simulink model "Thrustersim"  (R2018b)
settings: Solver=FixedStepAuto  StartTime=0.0  StopTime=100.0  FixedStep=.1  RelTol=1e-3
values from neighbouring files (symbols this model uses):
  R_2_t = [1 1 -1 -1; 1 -1 -1 1; 1 -1 1 -1; 1 1 1 1]    [Thruster_supprt.m]
libraries: simulink x3
settings Model: DataTypeOverride=Double  MinMaxOverflowLogging=ForceOff  Creator=Stefan's Laptop  LastModifiedBy=Stefan's Laptop

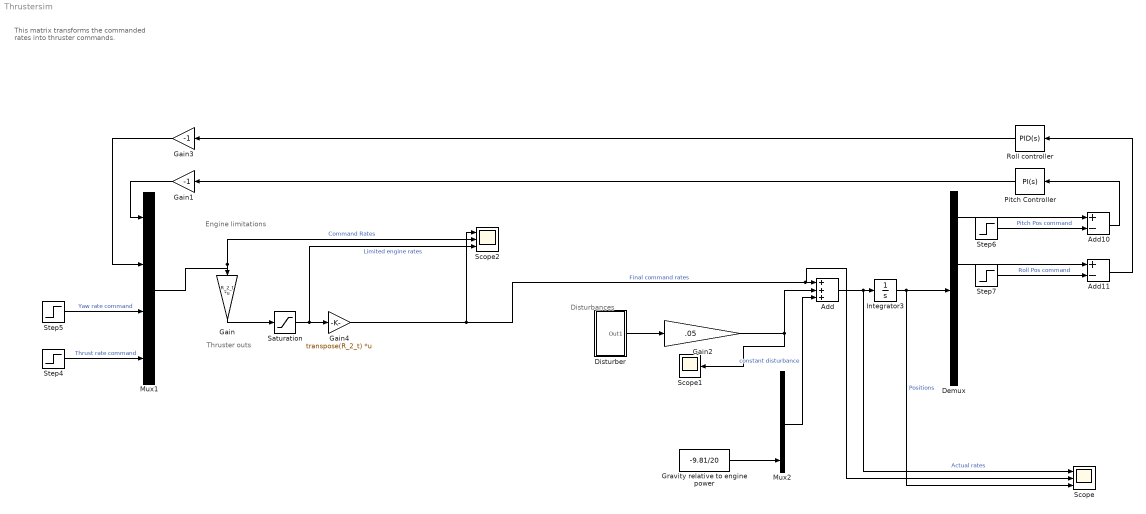
== system Thrustersim ==
  note: Engine limitations
  note: Disturbances
  note: Thruster outs
  note: This matrix transforms the commanded
      | rates into thruster commands.
  Add : Sum  Inputs=3
  Add10 : Sum  Inputs=+-
  Add11 : Sum  Inputs=+-
  Demux : Demux
  Disturber : Subsystem
  Gain : Gain  Gain=R_2_t  Multiplication=Matrix(K*u)
  Gain1 : Gain  Gain=-1
  Gain2 : Gain  Gain=.05
  Gain3 : Gain  Gain=-1
  Gain4 : Gain  Gain=transpose(R_2_t)  Multiplication=Matrix(K*u)
  Gravity relative to engine power : Constant  Value=-9.81/20
  Integrator3 : Integrator
  Mux1 : Mux
  Mux2 : Mux
  Pitch Controller : simulink/Continuous/PID Controller  Controller=PI  Form=Parallel  TimeDomain=Continuous-time  SampleTime=-1  IntegratorMethod=Forward Euler  FilterMethod=Forward Euler  ControllerParametersSource=internal  P=1  I=200  D=1  UseFilter=on  N=100  TunerSelectOption=Transfer Function Based (PID Tuner App)  InitialConditionSource=internal  InitialConditionForIntegrator=0  InitialConditionForFilter=0  DifferentiatorICPrevScaledInput=0  ExternalReset=none  TrackingMode=off  Kt=1  LimitOutput=off  UpperSaturationLimit=inf  LowerSaturationLimit=-inf  LinearizeAsGain=on  AntiWindupMode=none  Kb=1  POutMin=[]  POutMax=[]  IOutMin=[]  IOutMax=[]  DOutMin=[]  DOutMax=[]  NOutMin=[]  NOutMax=[]  SumOutMin=[]  SumOutMax=[]  SaturationOutMin=[]  SaturationOutMax=[]  PParamMin=[]  PParamMax=[]  IParamMin=[]  IParamMax=[]  DParamMin=[]  DParamMax=[]  NParamMin=[]  NParamMax=[]  KbParamMin=[]  KbParamMax=[]  KtParamMin=[]  KtParamMax=[]  KbOutMin=[]  KbOutMax=[]  KtOutMin=[]  KtOutMax=[]  IntegratorOutMin=[]  IntegratorOutMax=[]  FilterOutMin=[]  FilterOutMax=[]  SumI1OutMin=[]  SumI1OutMax=[]  SumI2OutMin=[]  SumI2OutMax=[]  SumI3OutMin=[]  SumI3OutMax=[]  SumI4OutMin=[]  SumI4OutMax=[]  SumDOutMin=[]  SumDOutMax=[]  DifferentiatorOutMin=[]  DifferentiatorOutMax=[]  FilterDiffOutCoefMin=[]  FilterDiffOutCoefMax=[]  ReciprocalOutMin=[]  ReciprocalOutMax=[]  SumDenOutMin=[]  SumDenOutMax=[]  SumNumOutMin=[]  SumNumOutMax=[]  DivideOutMin=[]  DivideOutMax=[]  IntegratorContinuousStateAttributes=''  IntegratorStateMustResolveToSignalObject=off  IntegratorRTWStateStorageClass=Auto  FilterContinuousStateAttributes=''  FilterStateMustResolveToSignalObject=off  FilterRTWStateStorageClass=Auto  ParallelPVariant=InternalParameters  IdealPVariant=Disabled  IVariant=InternalParameters  DVariant=Disabled  IntegratorVariant=Continuous  SatVariant=Disabled  AWVariant=Passthrough  PCopyVariant=Disabled  TRVariant=Disabled  FdbkBlocksVariant=Forward  IdealPFdbkVariant=Disabled  SatFdbkVariant=Disabled  DerivativeFilterVariant=Disabled  NVariant=Disabled  NCopyVariant=Disabled_SignalSpec  FilterICVariant=Disabled  IntegratorICVariant=InternalICs  ExternalResetVariant=Disabled  TRSumVariant=Passthrough  SumFdbkVariant=Disabled  SumVariant=Sum_PI
  Roll controller : simulink/Continuous/PID Controller  Controller=PID  Form=Parallel  TimeDomain=Continuous-time  SampleTime=-1  IntegratorMethod=Forward Euler  FilterMethod=Forward Euler  ControllerParametersSource=internal  P=1  I=1  D=0  UseFilter=on  N=100  TunerSelectOption=Transfer Function Based (PID Tuner App)  InitialConditionSource=internal  InitialConditionForIntegrator=0  InitialConditionForFilter=0  DifferentiatorICPrevScaledInput=0  ExternalReset=none  TrackingMode=off  Kt=1  LimitOutput=off  UpperSaturationLimit=inf  LowerSaturationLimit=-inf  LinearizeAsGain=on  AntiWindupMode=none  Kb=1  POutMin=[]  POutMax=[]  IOutMin=[]  IOutMax=[]  DOutMin=[]  DOutMax=[]  NOutMin=[]  NOutMax=[]  SumOutMin=[]  SumOutMax=[]  SaturationOutMin=[]  SaturationOutMax=[]  PParamMin=[]  PParamMax=[]  IParamMin=[]  IParamMax=[]  DParamMin=[]  DParamMax=[]  NParamMin=[]  NParamMax=[]  KbParamMin=[]  KbParamMax=[]  KtParamMin=[]  KtParamMax=[]  KbOutMin=[]  KbOutMax=[]  KtOutMin=[]  KtOutMax=[]  IntegratorOutMin=[]  IntegratorOutMax=[]  FilterOutMin=[]  FilterOutMax=[]  SumI1OutMin=[]  SumI1OutMax=[]  SumI2OutMin=[]  SumI2OutMax=[]  SumI3OutMin=[]  SumI3OutMax=[]  SumI4OutMin=[]  SumI4OutMax=[]  SumDOutMin=[]  SumDOutMax=[]  DifferentiatorOutMin=[]  DifferentiatorOutMax=[]  FilterDiffOutCoefMin=[]  FilterDiffOutCoefMax=[]  ReciprocalOutMin=[]  ReciprocalOutMax=[]  SumDenOutMin=[]  SumDenOutMax=[]  SumNumOutMin=[]  SumNumOutMax=[]  DivideOutMin=[]  DivideOutMax=[]  IntegratorContinuousStateAttributes=''  IntegratorStateMustResolveToSignalObject=off  IntegratorRTWStateStorageClass=Auto  FilterContinuousStateAttributes=''  FilterStateMustResolveToSignalObject=off  FilterRTWStateStorageClass=Auto  ParallelPVariant=InternalParameters  IdealPVariant=Disabled  IVariant=InternalParameters  DVariant=InternalParameters  IntegratorVariant=Continuous  SatVariant=Disabled  AWVariant=Passthrough  PCopyVariant=Disabled  TRVariant=Disabled  FdbkBlocksVariant=Forward  IdealPFdbkVariant=Disabled  SatFdbkVariant=Disabled  DerivativeFilterVariant=ContFilter  NVariant=InternalParameters  NCopyVariant=Disabled  FilterICVariant=InternalICsFilter  IntegratorICVariant=InternalICs  ExternalResetVariant=Disabled  TRSumVariant=Passthrough  SumFdbkVariant=Disabled  SumVariant=Sum_PID
  Saturation : Saturate  UpperLimit=1  LowerLimit=0
  Scope : Scope  NumInputPorts=3
  Scope1 : Scope
  Scope2 : Scope  NumInputPorts=3
  Step4 : Step  After=.5  SampleTime=0
  Step5 : Step  After=0  SampleTime=0
  Step6 : Step  SampleTime=0
  Step7 : Step  After=0  SampleTime=0
  wires:
  Step4/1 -> Mux1/4  "Thrust rate command"
  Pitch Controller/1 -> Gain1/1
  Roll controller/1 -> Gain3/1
  Mux1/1 -> Scope2/2, Gain/1  "Command Rates"
  Integrator3/1 -> Scope/3, Demux/1  "Positions"
  Step6/1 -> Add10/2  "Pitch Pos command"
  Demux/1 -> Add10/1
  Add10/1 -> Pitch Controller/1
  Demux/2 -> Add11/1
  Step7/1 -> Add11/2  "Roll Pos command"
  Add11/1 -> Roll controller/1
  Step5/1 -> Mux1/3  "Yaw rate command"
  Add/1 -> Scope/1, Integrator3/1  "Actual rates"
  Mux2/1 -> Add/3  "constant disturbance"
  Gravity relative to engine power/1 -> Mux2/4
  Gain2/1 -> Scope1/1, Add/2
  Disturber/1(Out1) -> Gain2/1
  Gain1/1 -> Mux1/1
  Gain3/1 -> Mux1/2
  Gain/1 -> Saturation/1
  Saturation/1 -> Scope2/3, Gain4/1  "Limited engine rates"
  Gain4/1 -> Scope2/1, Scope/2, Add/1  "Final command rates"

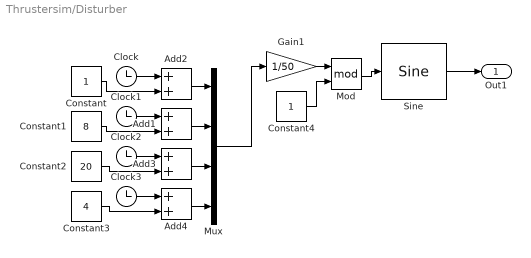
== system Thrustersim/Disturber ==
  Add{1..4} (4 alike) : Sum  Inputs=2
  Clock{,1..3} (4 alike) : Clock
  Constant : Constant
  Constant1 : Constant  Value=8
  Constant2 : Constant  Value=20
  Constant3 : Constant  Value=4
  Constant4 : Constant
  Gain1 : Gain  Gain=1/50
  Mod : Math  Operator=mod  SaturateOnIntegerOverflow=on
  Mux : Mux
  Sine : simulink/Lookup Tables/Sine  Formula=sin(2*pi*u)  NumDataPoints=100  OutputWordLength=16  InternalRulePriority=Speed
      settings: SourceProductName=Simulink
  Out1 : Outport
  wires:
  Clock/1 -> Add2/1
  Mux/1 -> Gain1/1
  Add4/1 -> Mux/4
  Clock3/1 -> Add4/1
  Mod/1 -> Sine/1
  Gain1/1 -> Mod/1
  Constant2/1 -> Add3/2
  Add1/1 -> Mux/2
  Clock2/1 -> Add3/1
  Add3/1 -> Mux/3
  Add2/1 -> Mux/1
  Constant3/1 -> Add4/2
  Clock1/1 -> Add1/1
  Constant1/1 -> Add1/2
  Constant/1 -> Add2/2
  Sine/1 -> Out1/1
  Constant4/1 -> Mod/2
